simulink library "PhaseDetectBtc"  (R2022b)
settings: Solver=VariableStepAuto  StartTime=0.0  StopTime=10.0  RelTol=1e-3
libraries: StateVar x4, RTC x2, FeaturePath x1, HandyTextFile x1
settings Model: Creator=kl13806  LastModifiedBy=kl13806
settings SolverCC: AlgebraicLoopSolver=TrustRegion
settings DebuggingCC: UnconnectedInputMsg=warning  UnconnectedOutputMsg=warning  UnconnectedLineMsg=warning  SFMachineParentedDataDiag=warning
settings ModelReferenceCC: EnableRefExpFcnMdlSchedulingChecks=on
settings RTWCC: DLArmComputeVersion=19.05

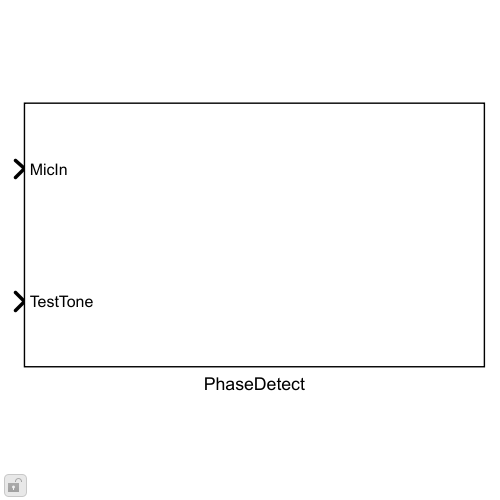
[thumbnail: Simulink's stored preview of the top-level diagram]
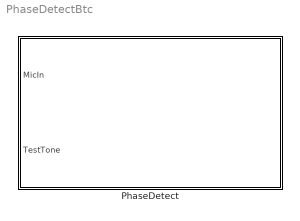
== system PhaseDetectBtc ==
  PhaseDetect : Subsystem  mask(Blocklib PhaseDetector){Config=[], FeatureName=PhaseDetector}
      mask prompts: Config "PhaseDetectConfig"; FeatureName "Feature path name:"
      mask init:
      | blkh=gcbh;
      | Config=BTConfig.Assert(blkh,Config);
      | Config.Validate();
      | BTConfig.InitSetFeatureIfPresent(blkh,'FeatureName');
      mask Callback Config: BTConfig.CallbackHideIfPresent(gcbh,{'FeatureName'});
      mask TypeOptions FeatureName: FeaturePath/FeatureName

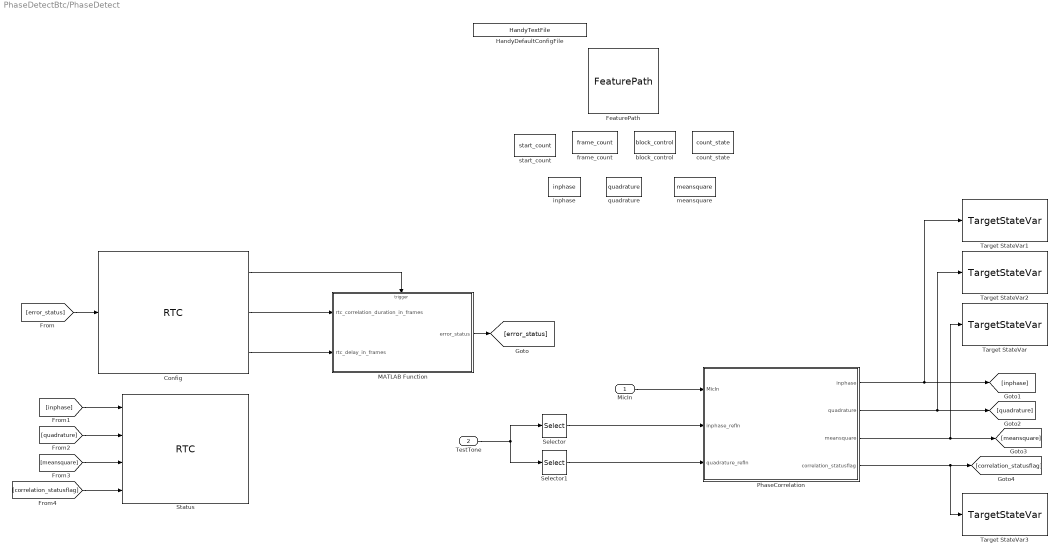
== system PhaseDetectBtc/PhaseDetect ==
  MicIn : Inport
  TestTone : Inport  Port=2
  Config : RTC/RTC  REQ_Priority=RTC_Mask.NormalPriority  RequestAtInit=off  EnableRequest=on  REQElemName1=correlation_duration_in_frames  REQElemType1=int32  REQElemWidth1=1  REQElemInitial1=[]  REQElemName2=delay_in_frames  REQElemType2=int32  REQElemWidth2=1  REQElemInitial2=[]  REQElemType3=uint32  REQElemWidth3=1  REQElemInitial3=[]  REQElemType4=uint32  REQElemWidth4=1  REQElemInitial4=[]  REQElemType5=uint32  REQElemWidth5=1  REQElemInitial5=[]  REQElemType6=uint32  REQElemWidth6=1  REQElemInitial6=[]  REQElemType7=uint32  REQElemWidth7=1  REQElemInitial7=[]  REQElemType8=uint32  REQElemWidth8=1  REQElemInitial8=[]  REQElemType9=uint32  REQElemWidth9=1  REQElemInitial9=[]  REQElemType10=uint32  REQElemWidth10=1  REQElemInitial10=[]  EnableResponse=on  EnableRSP_StatusIn=off  RSPElemName1=errStatus  RSPElemType1=uint32  RSPElemWidth1=1  RSPElemType2=uint32  RSPElemWidth2=1  RSPElemType3=uint32  RSPElemWidth3=1  RSPElemType4=uint32  RSPElemWidth4=1  RSPElemType5=uint32  RSPElemWidth5=1  RSPElemType6=uint32  RSPElemWidth6=1  RSPElemType7=uint32  RSPElemWidth7=1  RSPElemType8=uint32  RSPElemWidth8=1  RSPElemType9=uint32  RSPElemWidth9=1  RSPElemType10=uint32  RSPElemWidth10=1  EnableNotification=off  EnableNTF_PrepTrig=off  NTFElemType1=uint32  NTFElemWidth1=1  NTFElemType2=uint32  NTFElemWidth2=1  NTFElemType3=uint32  NTFElemWidth3=1  NTFElemType4=uint32  NTFElemWidth4=1  NTFElemType5=uint32  NTFElemWidth5=1  NTFElemType6=uint32  NTFElemWidth6=1  NTFElemType7=uint32  NTFElemWidth7=1  NTFElemType8=uint32  NTFElemWidth8=1  NTFElemType9=uint32  NTFElemWidth9=1  NTFElemType10=uint32  NTFElemWidth10=1  MaskMessageName=Config
  FeaturePath : FeaturePath/FeaturePath  FeatureName=PhaseDetector  IsGroup=off  GroupNumber=-1  IsModule=off  TriggerInit=[815 19 930 126]
  HandyDefaultConfigFile : HandyTextFile/HandyTextFile  TemplateSource=Config  FileSuffix=Init  OpenDialogOnLoad=off  UseThisBlockName=off  TheDefaultText=|  ShowInLibBrowser=on
      | % $(FILENAME) Setup model parameters for each "Init" callback (e.g. update diagram)
      | sample_rate_in_hertz = 44100;
      | frame_size = 32;
      | sysin_channel_count = 2;
  MATLAB Function : MATLAB Function  TreatAsAtomicUnit=on  mask{numMicIn=Config.NumMicIn}
  PhaseCorrelation : Subsystem
  Selector : Selector  NumberOfDimensions=2  InputPortWidth=3  IndexOptions=Select all,Index vector (dialog)  Indices=[1 2],1  OutputSizes=1,1
  Selector1 : Selector  NumberOfDimensions=2  InputPortWidth=3  IndexOptions=Select all,Index vector (dialog)  Indices=[1 2],2  OutputSizes=1,1
  Status : RTC/RTC  REQ_Priority=RTC_Mask.NormalPriority  RequestAtInit=off  EnableRequest=off  REQElemType1=single  REQElemWidth1=1  REQElemInitial1=[]  REQElemType2=single  REQElemWidth2=1  REQElemInitial2=[]  REQElemType3=single  REQElemWidth3=1  REQElemInitial3=[]  REQElemType4=uint32  REQElemWidth4=1  REQElemInitial4=[]  REQElemType5=uint32  REQElemWidth5=1  REQElemInitial5=[]  REQElemType6=uint32  REQElemWidth6=1  REQElemInitial6=[]  REQElemType7=uint32  REQElemWidth7=1  REQElemInitial7=[]  REQElemType8=uint32  REQElemWidth8=1  REQElemInitial8=[]  REQElemType9=uint32  REQElemWidth9=1  REQElemInitial9=[]  REQElemType10=uint32  REQElemWidth10=1  REQElemInitial10=[]  EnableResponse=on  EnableRSP_StatusIn=off  RSPElemName1=inphase  RSPElemType1=single  RSPElemWidth1=Config.NumMicIn  RSPElemName2=quadrature  RSPElemType2=single  RSPElemWidth2=Config.NumMicIn  RSPElemName3=meansquare  RSPElemType3=single  RSPElemWidth3=Config.NumMicIn  RSPElemName4=correlation_statusflag  RSPElemType4=int32  RSPElemWidth4=1  RSPElemType5=uint32  RSPElemWidth5=1  RSPElemType6=uint32  RSPElemWidth6=1  RSPElemType7=uint32  RSPElemWidth7=1  RSPElemType8=uint32  RSPElemWidth8=1  RSPElemType9=uint32  RSPElemWidth9=1  RSPElemType10=uint32  RSPElemWidth10=1  EnableNotification=off  EnableNTF_PrepTrig=off  NTFElemType1=uint32  NTFElemWidth1=1  NTFElemType2=uint32  NTFElemWidth2=1  NTFElemType3=uint32  NTFElemWidth3=1  NTFElemType4=uint32  NTFElemWidth4=1  NTFElemType5=uint32  NTFElemWidth5=1  NTFElemType6=uint32  NTFElemWidth6=1  NTFElemType7=uint32  NTFElemWidth7=1  NTFElemType8=uint32  NTFElemWidth8=1  NTFElemType9=uint32  NTFElemWidth9=1  NTFElemType10=uint32  NTFElemWidth10=1  MaskMessageName=Status
  Target StateVar : StateVar/TargetStateVar  TriggerInit=[1425 436 1565 504]  TspName=Mic_rms  StateName=Mic_rms  UseSameName=on  IfdefMacro=[]
  Target StateVar1 : StateVar/TargetStateVar  TriggerInit=[1425 266 1565 334]  TspName=Xcorr_inphase  StateName=Xcorr_inphase  UseSameName=on  IfdefMacro=[]
  Target StateVar2 : StateVar/TargetStateVar  TriggerInit=[1425 351 1565 419]  TspName=Xcorr_quad  StateName=Xcorr_quad  UseSameName=on  IfdefMacro=[]
  Target StateVar3 : StateVar/TargetStateVar  TriggerInit=[1425 746 1565 814]  TspName=MeasureInProgress  StateName=MeasureInProgress  UseSameName=on  IfdefMacro=[]
  block_control : DataStoreMemory  DataStoreName=block_control  ShowAdditionalParam=off  OutDataTypeStr=int32
  count_state : DataStoreMemory  DataStoreName=count_state  InitialValue=Config.InitialFrameCount  ShowAdditionalParam=off  OutDataTypeStr=int32
  frame_count : DataStoreMemory  DataStoreName=frame_count  InitialValue=Config.InitialFrameCount  ShowAdditionalParam=off  OutDataTypeStr=int32
  inphase : DataStoreMemory  DataStoreName=inphase  InitialValue=zeros(Config.NumMicIn,1)  ShowAdditionalParam=off  OutDataTypeStr=single
  meansquare : DataStoreMemory  DataStoreName=meansquare  InitialValue=zeros(Config.NumMicIn,1)  ShowAdditionalParam=off  OutDataTypeStr=single
  quadrature : DataStoreMemory  DataStoreName=quadrature  InitialValue=zeros(Config.NumMicIn,1)  ShowAdditionalParam=off  OutDataTypeStr=single
  start_count : DataStoreMemory  DataStoreName=start_count  InitialValue=Config.InitialStartCount  ShowAdditionalParam=off  OutDataTypeStr=int32
  wires:
  PhaseCorrelation/1(inphase) -> [inphase], Target StateVar1/1
  PhaseCorrelation/3(meansquare) -> [meansquare], Target StateVar/1
  Config/2 -> MATLAB Function/1(rtc_correlation_duration_in_frames)
  [inphase] -> Status/1
  Selector1/1 -> PhaseCorrelation/3(quadrature_refIn)
  Config/1 -> MATLAB Function/Trigger
  [error_status] -> Config/1
  PhaseCorrelation/2(quadrature) -> [quadrature], Target StateVar2/1
  Selector/1 -> PhaseCorrelation/2(inphase_refIn)
  PhaseCorrelation/4(correlation_statusflag) -> [correlation_statusflag], Target StateVar3/1
  [quadrature] -> Status/2
  [meansquare] -> Status/3
  MicIn/1 -> PhaseCorrelation/1(MicIn)
  MATLAB Function/1(error_status) -> [error_status]
  Config/3 -> MATLAB Function/2(rtc_delay_in_frames)
  [correlation_statusflag] -> Status/4
  TestTone/1 -> Selector1/1, Selector/1

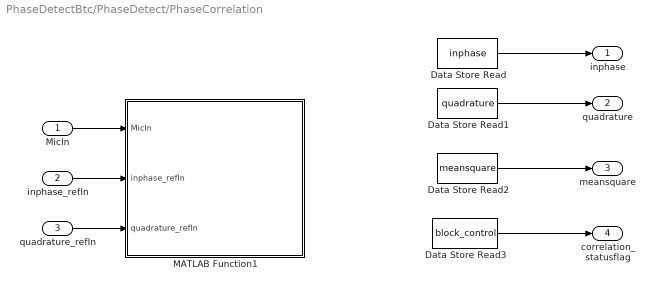
== system PhaseDetectBtc/PhaseDetect/PhaseCorrelation ==
  MicIn : Inport
  inphase_refIn : Inport  Port=2
  quadrature_refIn : Inport  Port=3
  Data Store Read : DataStoreRead  DataStoreName=inphase  IndexOptions=Index vector (dialog)  Indices=1  OutputSizes=1
  Data Store Read1 : DataStoreRead  DataStoreName=quadrature  IndexOptions=Index vector (dialog)  Indices=1  OutputSizes=1
  Data Store Read2 : DataStoreRead  DataStoreName=meansquare  IndexOptions=Index vector (dialog)  Indices=1  OutputSizes=1
  Data Store Read3 : DataStoreRead  DataStoreName=block_control  IndexOptions=Index vector (dialog)  Indices=1  OutputSizes=1
  MATLAB Function1 : MATLAB Function  TreatAsAtomicUnit=on  mask{numMicIn=Config.NumMicIn, frameSize=Config.FrameSize}
  inphase : Outport
  quadrature : Outport  Port=2
  meansquare : Outport  Port=3
  correlation_statusflag : Outport  Port=4
  wires:
  Data Store Read1/1 -> quadrature/1
  Data Store Read2/1 -> meansquare/1
  Data Store Read3/1 -> correlation_statusflag/1
  Data Store Read/1 -> inphase/1
  inphase_refIn/1 -> MATLAB Function1/2(inphase_refIn)
  MicIn/1 -> MATLAB Function1/1(MicIn)
  quadrature_refIn/1 -> MATLAB Function1/3(quadrature_refIn)

== matlab function PhaseDetectBtc/PhaseDetect/MATLAB Function ==
  data: rtc_correlation_duration_in_frames input int32 size=1; error_status output uint32 size=1; rtc_delay_in_frames input int32 size=1; inphase data_store_memory; quadrature data_store_memory; meansquare data_store_memory; block_control data_store_memory; frame_count data_store_memory; count_state data_store_memory; numMicIn parameter double size=1; start_count data_store_memory
  events: trigger input FUNCTION_CALL_EVENT
function error_status = phaseDetectorconfig(rtc_correlation_duration_in_frames,rtc_delay_in_frames, numMicIn)
    %#codegen
    % datastore memory to control the audio processing logic:
    global inphase;
    global quadrature;
    global meansquare;
    global start_count;
    global frame_count;
    global block_control;
    global count_state;  
    % Error status   
    error_status = uint32(0);  
    % Error check
    % rtc_correlation_duration_in_frames and rtc_delay_in_frames should be positive
    if((rtc_correlation_duration_in_frames < 0) || (rtc_delay_in_frames < 0)) 
        error_status = uint32(1);      
    else
        %turn off
        if(block_control~=0)
            block_control = int32(0);
        end
        % load the count values
        start_count   = rtc_correlation_duration_in_frames;
        frame_count   = rtc_delay_in_frames + rtc_correlation_duration_in_frames;
        count_state   = frame_count;
        % clear the states
        inphase      = single(zeros(numMicIn,1));
        quadrature   = single(zeros(numMicIn,1));
        meansquare   = single(zeros(numMicIn,1));  
        % turn on
        block_control = int32(1);
    end

== matlab function PhaseDetectBtc/PhaseDetect/PhaseCorrelation/MATLAB Function1 ==
  data: MicIn input single size=[Config.FrameSize Config.NumMicIn]; inphase_refIn input single size=[Config.FrameSize 1]; quadrature_refIn input single size=[Config.FrameSize 1]; inphase data_store_memory; meansquare data_store_memory; quadrature data_store_memory; start_count data_store_memory; frame_count data_store_memory; block_control data_store_memory; count_state data_store_memory; numMicIn parameter single size=1; frameSize parameter
function phase_correlation(MicIn, inphase_refIn,quadrature_refIn, numMicIn, frameSize)
    %#codegen
    % datastore memory to control the audio processing logic:
    global inphase;
    global quadrature;
    global meansquare;
    global start_count;
    global frame_count;
    global block_control;
    global count_state;
    
  if (block_control ~= 0)    % Calculate correlations when blockControl ~= 0
      count_state = count_state - 1;
      if (count_state >= start_count)
          return;
      end

      inphase = inphase + MicIn(:,1:numMicIn)' * inphase_refIn(:,1);            % correlation between inputs and in-phase reference
      quadrature = quadrature + MicIn(:,1:numMicIn)' * quadrature_refIn(:,1);   % correlation between inputs and quadrature reference

      for i=1:numMicIn
          meansquare(i) = meansquare(i) + MicIn(:,i)' * MicIn(:,i);
      end

      if (count_state <= 0)
          count_state = frame_count;                 % reload counter
          scaling = single(frameSize * start_count);
          inphase = inphase / scaling;             % normalization
          quadrature = quadrature / scaling;
          meansquare = meansquare / scaling;
          block_control = int32(0);
      end
  end
